simulink model "Antriebsstrangmodell_V1_4_n5_WHasym"  (R2019a)
(part 3 of 5)

  R_toBR_a(2.2)/LConn1 -- T_SH_a(2)/LConn1 -- C_SH_a(2)/LConn1 -- R_toBR_a(2.1)/RConn1 -- R_toRYO3(2)/RConn1
  R_toRSLTO(2)/RConn1 -- T_RYO(2)/LConn1 -- C_RYO(2)/LConn1 -- R_toSH(2)/LConn1 -- PV_RYO(2)/LConn1
  R_toRSL2(2)/RConn1 -- R_toRTO(2)/LConn1
  Thermal Reference32/LConn1 -- PV_RSL(2)/RConn2
  Thermal Reference33/LConn1 -- PV_RTO(2)/RConn2
  R_toRAGP(2)/LConn1 -- air-gap convection AGP to RSL (2)/RConn1
  Thermal Reference31/LConn1 -- PV_RYO(2)/RConn2
  R_toRAGP2(2)/LConn1 -- air-gap convection AGP to RTO (2)/RConn1
  R_toRTO(3)/RConn1 -- R_toRAGP(3)/RConn1 -- T_RSL(3)/LConn1 -- C_RSL(3)/LConn1 -- PV_RSL(3)/LConn1 -- R_toER(3.2)/LConn1 -- R_toER(3.1)/RConn1 -- R_toRYO(3)/LConn1
  C_RTO(3)/LConn1 -- T_RTO(3)/LConn1 -- PV_RTO(3)/LConn1 -- R_toRYO2(3)/LConn1 -- R_toRAGP2(3)/RConn1 -- R_toRSL2(3)/LConn1
  R_toRYO2(3)/RConn1 -- R_toRYO(3)/RConn1 -- R_toRSLTO(3)/LConn1
  R_toRSLTO(3)/RConn1 -- T_RYO(3)/LConn1 -- C_RYO(3)/LConn1 -- R_toSH(3)/LConn1 -- PV_RYO(3)/LConn1
  R_toRSL2(3)/RConn1 -- R_toRTO(3)/LConn1
  Thermal Reference35/LConn1 -- PV_RSL(3)/RConn2
  Thermal Reference36/LConn1 -- PV_RTO(3)/RConn2
  R_toRAGP(3)/LConn1 -- air-gap convection AGP to RSL (3)/RConn1
  Thermal Reference34/LConn1 -- PV_RYO(3)/RConn2
  R_toRAGP2(3)/LConn1 -- air-gap convection AGP to RTO (3)/RConn1
  R_toRTO(4)/RConn1 -- R_toRAGP(4)/RConn1 -- T_RSL(4)/LConn1 -- C_RSL(4)/LConn1 -- PV_RSL(4)/LConn1 -- R_toER(4.2)/LConn1 -- R_toER(4.1)/RConn1 -- R_toRYO(4)/LConn1
  C_RTO(4)/LConn1 -- T_RTO(4)/LConn1 -- PV_RTO(4)/LConn1 -- R_toRYO2(4)/LConn1 -- R_toRAGP2(4)/RConn1 -- R_toRSL2(4)/LConn1
  R_toRYO2(4)/RConn1 -- R_toRYO(4)/RConn1 -- R_toRSLTO(4)/LConn1
  R_toBR_a(4.2)/LConn1 -- T_SH_a(4)/LConn1 -- C_SH_a(4)/LConn1 -- R_toBR_a(4.1)/RConn1 -- R_toRYO3(4)/RConn1
  R_toRSLTO(4)/RConn1 -- T_RYO(4)/LConn1 -- C_RYO(4)/LConn1 -- R_toSH(4)/LConn1 -- PV_RYO(4)/LConn1
  R_toRSL2(4)/RConn1 -- R_toRTO(4)/LConn1
  Thermal Reference38/LConn1 -- PV_RSL(4)/RConn2
  Thermal Reference39/LConn1 -- PV_RTO(4)/RConn2
  R_toRAGP(4)/LConn1 -- air-gap convection AGP to RSL (4)/RConn1
  Thermal Reference37/LConn1 -- PV_RYO(4)/RConn2
  R_toRAGP2(4)/LConn1 -- air-gap convection AGP to RTO (4)/RConn1
  R_toRTO(5)/RConn1 -- R_toRAGP(5)/RConn1 -- T_RSL(5)/LConn1 -- C_RSL(5)/LConn1 -- PV_RSL(5)/LConn1 -- R_toER(5.2)/LConn1 -- R_toER(5.1)/RConn1 -- R_toRYO(5)/LConn1
  C_RTO(5)/LConn1 -- T_RTO(5)/LConn1 -- PV_RTO(5)/LConn1 -- R_toRYO2(5)/LConn1 -- R_toRAGP2(5)/RConn1 -- R_toRSL2(5)/LConn1
  R_toRYO(5)/RConn1 -- R_toRYO2(5)/RConn1 -- R_toRSLTO(5)/LConn1
  R_toBR_a(5.2)/LConn1 -- T_SH_a(5)/LConn1 -- C_SH_a(5)/LConn1 -- R_toBR_a(5.1)/RConn1 -- R_toRYO3(5)/RConn1
  R_toRSLTO(5)/RConn1 -- T_RYO(5)/LConn1 -- C_RYO(5)/LConn1 -- R_toSH(5)/LConn1 -- PV_RYO(5)/LConn1
  R_toRSL2(5)/RConn1 -- R_toRTO(5)/LConn1
  Thermal Reference41/LConn1 -- PV_RSL(5)/RConn2
  Thermal Reference42/LConn1 -- PV_RTO(5)/RConn2
  R_toRAGP(5)/LConn1 -- air-gap convection AGP to RSL (5)/RConn1
  Thermal Reference40/LConn1 -- PV_RYO(5)/RConn2
  R_toRAGP2(5)/LConn1 -- air-gap convection AGP to RTO (5)/RConn1
  R_toER(2.1)/LConn1 -- R_toER(1.2)/RConn1
  R_toER(2.2)/RConn1 -- R_toER(3.1)/LConn1
  R_toER(3.2)/RConn1 -- R_toER(4.1)/LConn1
  R_toER(4.2)/RConn1 -- R_toER(5.1)/LConn1
  C_ER(2)/LConn1 -- T_ER(2)/LConn1 -- R_toIA4(2)/RConn1 -- PV_ER(2)/LConn1 -- R_toIA3(2)/LConn1 -- R_toRSL(2.2)/LConn1 -- R_toRSL(2.1)/RConn1
  Thermal Reference6/LConn1 -- PV_ER(2)/RConn2
  C_ER(1)/LConn1 -- T_ER(1)/LConn1 -- R_toIA4(1)1/RConn1 -- R_toRSL(1.2)/LConn1 -- R_toIA3(1)/LConn1 -- PV_ER(1)/LConn1 -- R_toRSL(1.1)/RConn1
  Thermal Reference43/LConn1 -- PV_ER(1)/RConn2
  Thermal Reference5/LConn1 -- T_ER(1)/RConn1
  R_toEC_p(1.2)/RConn1 -- R_toEC_a(1.1)/LConn1
  R_toEC_p(2.2)/LConn1 -- C_HO_p(2)/LConn1 -- T_HO_p(2)/LConn1 -- R_toEC_p(2.1)/RConn1 -- R_toIA5(2)/LConn1 -- R_toWC_p(2)/RConn1
  R_toEC_p(2.1)/LConn1 -- R_toEC_a(5.2)/RConn1
  R_toHO2(2)/LConn1 -- R_toEC_p(2.2)/RConn1
  R_toBR2(2)/LConn1 -- T_EC(2)/LConn1 -- C_EC(2)/LConn1 -- R_toHO2(2)/RConn1 -- R_toIA7(2)/RConn1
  R_toBR2(1)/LConn1 -- R_toHO2(1)/RConn1 -- C_EC(1)/LConn1 -- R_toIA7(1)/LConn1 -- T_EC(1)/LConn1
  R_toHO2(1)/LConn1 -- R_toEC_p(1.1)/LConn1
  Thermal Reference4/LConn1 -- PV_BR(1.1)/RConn2
  R_toBR_p(1.2)/RConn1 -- R_toBR_a(1.1)/LConn1
  R_contactBR(1)/RConn1 -- PV_BR(1.2)/LConn1 -- R_toBR_p(1.1)/LConn1 -- Solver Configuration/RConn1
  R_toBR_a(2.2)/RConn1 -- R_toBR_a(3.1)/LConn1
  R_toBR_a(2.1)/LConn1 -- R_toBR_a(1.2)/RConn1
  R_toBR_a(3.2)/RConn1 -- R_toBR_a(4.1)/LConn1
  R_toBR_a(4.2)/RConn1 -- R_toBR_a(5.1)/LConn1
  R_toBR_a(5.2)/RConn1 -- R_toBR_p(2.1)/LConn1
  inner air convection EC to inner air (1)/LConn1 -- inner air convection WH to inner air (1.2)/LConn1 -- inner air convection HO to inner air (1)/LConn1 -- inner air convection WH to inner air (1.1)/LConn1 -- inner air convection WH to inner air (1.3)/LConn1 -- inner air convection ER to inner air (1.1)/LConn1 -- inner air convection SH to inner air (1)/LConn1 -- T_IA(1)/LConn1 -- PV_IA(1)/LConn1 -- inner air convection ER to inner air (1.2)/LConn1 -- inner air convection ER to inner air (1.3)/LConn1
  inner air convection EC to inner air (1)/LConn2 -- inner air convection HO to inner air (1)/LConn2 -- inner air convection WH to inner air (1.2)/LConn2 -- inner air convection WH to inner air (1.1)/LConn2 -- inner air convection WH to inner air (1.3)/LConn2 -- Simulink-PS Converter2/RConn1 -- inner air convection ER to inner air (1.1)/LConn2 -- inner air convection ER to inner air (1.2)/LConn2 -- inner air convection SH to inner air (1)/LConn2 -- inner air convection ER to inner air (1.3)/LConn2 -- inner air convection HO to inner air (2)/LConn2 -- inner air convection WH to inner air (2.2)/LConn2 -- inner air convection WH to inner air (2.1)/LConn2 -- inner air convection WH to inner air (2.3)/LConn2 -- inner air convection SH to inner air (2)/LConn2 -- inner air convection ER to inner air (2.2)/LConn2 -- inner air convection ER to inner air (2.1)/LConn2 -- inner air convection ER to inner air (2.3)/LConn2 -- inner air convection EC to inner air (2)/LConn2
  PV_ER(2)/RConn1 -- Simulink-PS Converter14/RConn1
  Simulink-PS Converter19/RConn1 -- PV_BR(2.2)/RConn1 -- PV_BR(2.1)/RConn1
  Simulink-PS Converter9/RConn1 -- PV_BR(1.2)/RConn1 -- PV_BR(1.1)/RConn1
  Thermal Reference45/LConn1 -- T_SSL(5)/RConn1
  Thermal Reference46/LConn1 -- T_SSL(4)/RConn1
  R_toSSL(2.2)/RConn1 -- inner air convection WH to inner air (2.1)/RConn1
  C_WH(2)/LConn1 -- T_WH(2)/LConn1 -- R_toIA2(2)/LConn1 -- PV_WH(2)/LConn1 -- R_toSSL(2.2)/LConn1 -- R_toIA(2)/RConn1 -- R_toSSL(2.1)/RConn1
  R_toWH(1.1)/LConn1 -- R_toSSL(1.2)/RConn1
  R_contactHO (1)/RConn1 -- R_toHO(1)/LConn1
  R_toHO(2)/LConn1 -- R_contactHO (2)/RConn1
  R_toHO(5)/LConn1 -- R_contactHO (5)/RConn1
  R_toRSL(1.1)/LConn1 -- inner air convection ER to inner air (1.1)/RConn1
  R_toER(1.1)/LConn1 -- R_toRSL(1.2)/RConn1
  R_toRSL(2.1)/LConn1 -- R_toER(5.2)/RConn1
  R_toRSL(2.2)/RConn1 -- inner air convection ER to inner air (2.1)/RConn1
  inner air convection ER to inner air (1.2)/RConn1 -- R_toIA3(1)/RConn1
  inner air convection ER to inner air (1.3)/RConn1 -- R_toIA4(1)1/LConn1
  inner air convection ER to inner air (2.2)/RConn1 -- R_toIA3(2)/RConn1
  inner air convection ER to inner air (2.3)/RConn1 -- R_toIA4(2)/LConn1
  air-gap convection AGP to RSL (2)/LConn1 -- air-gap convection AGP to SSL (2)/LConn1 -- T_AGP(2)/LConn1 -- air-gap convection AGP to STO (2)/LConn1 -- PV_AGP(2)/LConn1 -- air-gap convection AGP to RTO (2)/LConn1
  air-gap convection AGP to RSL (4)/LConn1 -- air-gap convection AGP to SSL (4)/LConn1 -- T_AGP(4)/LConn1 -- air-gap convection AGP to STO (4)/LConn1 -- PV_AGP(4)/LConn1 -- air-gap convection AGP to RTO (4)/LConn1
  air-gap convection AGP to STO (5)/LConn1 -- PV_AGP(5)/LConn1 -- T_AGP(5)/LConn1 -- air-gap convection AGP to RSL (5)/LConn1 -- air-gap convection AGP to SSL (5)/LConn1 -- air-gap convection AGP to RTO (5)/LConn1
  Thermal Reference44/LConn1 -- PV_AGP(2)/RConn2
  Thermal Reference47/LConn1 -- PV_AGP(3)/RConn2
  Thermal Reference48/LConn1 -- PV_AGP(4)/RConn2
  Thermal Reference49/LConn1 -- PV_AGP(5)/RConn2
  R_toEC_p(1.2)/LConn1 -- R_toIA5(1)/LConn1 -- R_toWC_p(1)/RConn1 -- C_HO_p(1)/LConn1 -- T_HO_p(1)/LConn1 -- R_toEC_p(1.1)/RConn1
  inner air convection WH to inner air (2.2)/RConn1 -- R_toIA(2)/LConn1
  R_toIA2(2)/RConn1 -- inner air convection WH to inner air (2.3)/RConn1
  R_toIA2(1)/RConn1 -- inner air convection WH to inner air (1.3)/RConn1
  R_toSSL(1.1)/LConn1 -- inner air convection WH to inner air (1.1)/RConn1
  inner air convection WH to inner air (1.2)/RConn1 -- R_toIA(1)/LConn1
  Convection HO to coolant (1)/LConn1 -- R_toWC_p(1)/LConn1
  Convection HO to coolant (7)/LConn1 -- R_toWC_p(2)/LConn1
  R_toIA5(1)/RConn1 -- inner air convection HO to inner air (1)/RConn1
  inner air convection HO to inner air (2)/RConn1 -- R_toIA5(2)/RConn1
  C_SH_a(1)/LConn1 -- R_toBR_a(1.2)/LConn1 -- R_toBR_a(1.1)/RConn1 -- R_toRYO3(1)/RConn1 -- T_SH_a(1)/LConn1
  R_toBR_a(3.2)/LConn1 -- T_SH_a(3)/LConn1 -- C_SH_a(3)/LConn1 -- R_toBR_a(3.1)/RConn1 -- R_toRYO3(3)/RConn1
  R_toIA6(1)/LConn1 -- inner air convection SH to inner air (1)/RConn1
  R_toIA6(1)/RConn1 -- C_SH_p(1)/LConn1 -- R_toBR_p(1.2)/LConn1 -- T_SH_p(1)/LConn1 -- R_toBR_p(1.1)/RConn1
  R_toIA6(2)/RConn1 -- T_SH_p(2)/LConn1 -- R_toBR_p(2.2)/LConn1 -- R_toBR_p(2.1)/RConn1 -- C_SH_p(2)/LConn1
  R_toIA6(2)/LConn1 -- inner air convection SH to inner air (2)/RConn1
  Thermal Reference50/LConn1 -- PV_BR(1.2)/RConn2
  PV_BR(1.1)/LConn1 -- R_toBR2(1)/RConn1 -- R_contactBR(1)/LConn1
  Thermal Reference51/LConn1 -- PV_BR(2.2)/RConn2
  R_toBR2(2)/RConn1 -- PV_BR(2.1)/LConn1 -- R_contactBR(2)/LConn1
  R_toIA7(1)/RConn1 -- inner air convection EC to inner air (1)/RConn1
  R_toIA7(2)/LConn1 -- inner air convection EC to inner air (2)/RConn1
  Thermal Reference53/LConn1 -- T_SSL(1)/RConn1
  Thermal Reference54/LConn1 -- T_SSL(2)/RConn1
  Simulink-PS Converter32/RConn1 -- PV_RYO(5)/RConn1
  PV_RYO(4)/RConn1 -- Simulink-PS Converter31/RConn1
  PV_RYO(3)/RConn1 -- Simulink-PS Converter30/RConn1
  PV_RYO(2)/RConn1 -- Simulink-PS Converter29/RConn1
  PV_RYO(1)/RConn1 -- Simulink-PS Converter16/RConn1
  Thermal Reference55/LConn1 -- T_RYO(1)/RConn1
  Thermal Reference56/LConn1 -- T_RYO(2)/RConn1
  Thermal Reference57/LConn1 -- T_RYO(3)/RConn1
  Thermal Reference58/LConn1 -- T_RYO(4)/RConn1
  Thermal Reference59/LConn1 -- T_RYO(5)/RConn1
  PS-Simulink Converter11/LConn1 -- T_RYO(5)/RConn2
  PS-Simulink Converter12/LConn1 -- T_RYO(4)/RConn2
  PS-Simulink Converter13/LConn1 -- T_RYO(3)/RConn2
  PS-Simulink Converter14/LConn1 -- T_RYO(2)/RConn2
  PS-Simulink Converter15/LConn1 -- T_RYO(1)/RConn2
  Simulink-PS Converter37/RConn1 -- PV_RTO(5)/RConn1
  Simulink-PS Converter36/RConn1 -- PV_RTO(4)/RConn1
  Simulink-PS Converter35/RConn1 -- PV_RTO(3)/RConn1
  Simulink-PS Converter34/RConn1 -- PV_RTO(2)/RConn1
  Simulink-PS Converter33/RConn1 -- PV_RTO(1)/RConn1
  Thermal Reference60/LConn1 -- T_RTO(1)/RConn1
  Thermal Reference61/LConn1 -- T_RTO(2)/RConn1
  Thermal Reference62/LConn1 -- T_RTO(3)/RConn1
  Thermal Reference63/LConn1 -- T_RTO(4)/RConn1
  Thermal Reference64/LConn1 -- T_RTO(5)/RConn1
  PS-Simulink Converter16/LConn1 -- T_RTO(5)/RConn2
  PS-Simulink Converter17/LConn1 -- T_RTO(4)/RConn2
  PS-Simulink Converter18/LConn1 -- T_RTO(3)/RConn2
  PS-Simulink Converter19/LConn1 -- T_RTO(2)/RConn2
  PS-Simulink Converter20/LConn1 -- T_RTO(1)/RConn2
  Simulink-PS Converter41/RConn1 -- PV_RSL(5)/RConn1
  Simulink-PS Converter40/RConn1 -- PV_RSL(4)/RConn1
  Simulink-PS Converter39/RConn1 -- PV_RSL(3)/RConn1
  Simulink-PS Converter38/RConn1 -- PV_RSL(2)/RConn1
  Simulink-PS Converter18/RConn1 -- PV_RSL(1)/RConn1
  Thermal Reference65/LConn1 -- T_RSL(2)/RConn1
  Thermal Reference66/LConn1 -- T_RSL(1)/RConn1
  Thermal Reference67/LConn1 -- T_RSL(4)/RConn1
  Thermal Reference68/LConn1 -- T_RSL(5)/RConn1
  PS-Simulink Converter21/LConn1 -- T_RSL(5)/RConn2
  PS-Simulink Converter22/LConn1 -- T_RSL(4)/RConn2
  PS-Simulink Converter23/LConn1 -- T_RSL(3)/RConn2
  PS-Simulink Converter24/LConn1 -- T_RSL(2)/RConn2
  T_RSL(1)/RConn2 -- PS-Simulink Converter25/LConn1
  Simulink-PS Converter13/RConn1 -- PV_ER(1)/RConn1
  PS-Simulink Converter5/LConn1 -- T_ER(2)/RConn2
  PS-Simulink Converter26/LConn1 -- T_ER(1)/RConn2
  Simulink-PS Converter6/RConn1 -- air-gap convection AGP to RSL (5)/LConn2 -- air-gap convection AGP to RTO (5)/LConn2 -- air-gap convection AGP to RSL (4)/LConn2 -- air-gap convection AGP to RTO (4)/LConn2 -- air-gap convection AGP to RSL (3)/LConn2 -- air-gap convection AGP to RTO (3)/LConn2 -- air-gap convection AGP to RSL (2)/LConn2 -- air-gap convection AGP to RTO (2)/LConn2 -- air-gap convection AGP to RSL (1)/LConn2 -- air-gap convection AGP to RTO (1)/LConn2 -- air-gap convection AGP to STO (1)/LConn2 -- air-gap convection AGP to SSL (2)/LConn2 -- air-gap convection AGP to STO (3)/LConn2 -- air-gap convection AGP to SSL (4)/LConn2 -- air-gap convection AGP to STO (5)/LConn2 -- air-gap convection AGP to SSL (5)/LConn2 -- air-gap convection AGP to STO (4)/LConn2 -- air-gap convection AGP to SSL (3)/LConn2 -- air-gap convection AGP to STO (2)/LConn2 -- air-gap convection AGP to SSL (1)/LConn2
  Thermal Reference69/LConn1 -- T_AGP(1)/RConn1
  Thermal Reference70/LConn1 -- T_AGP(2)/RConn1
  Thermal Reference71/LConn1 -- T_AGP(3)/RConn1
  Thermal Reference72/LConn1 -- T_AGP(4)/RConn1
  Thermal Reference73/LConn1 -- T_AGP(5)/RConn1
  PS-Simulink Converter6/LConn1 -- T_AGP(5)/RConn2
  PS-Simulink Converter27/LConn1 -- T_AGP(4)/RConn2
  PS-Simulink Converter29/LConn1 -- T_AGP(2)/RConn2
  PS-Simulink Converter28/LConn1 -- T_AGP(3)/RConn2
  T_AGP(1)/RConn2 -- PS-Simulink Converter30/LConn1
  Simulink-PS Converter12/RConn1 -- PV_AGP(1)/RConn1
  Simulink-PS Converter42/RConn1 -- PV_AGP(2)/RConn1
  PV_AGP(3)/RConn1 -- Simulink-PS Converter43/RConn1
  PV_AGP(4)/RConn1 -- Simulink-PS Converter44/RConn1
  PV_AGP(5)/RConn1 -- Simulink-PS Converter45/RConn1
  inner air convection EC to inner air (2)/LConn1 -- inner air convection HO to inner air (2)/LConn1 -- inner air convection WH to inner air (2.2)/LConn1 -- inner air convection WH to inner air (2.1)/LConn1 -- inner air convection WH to inner air (2.3)/LConn1 -- inner air convection ER to inner air (2.1)/LConn1 -- T_IA(2)/LConn1 -- inner air convection SH to inner air (2)/LConn1 -- PV_IA(2)/LConn1 -- inner air convection ER to inner air (2.2)/LConn1 -- inner air convection ER to inner air (2.3)/LConn1
  Thermal Reference52/LConn1 -- T_WH(1)/RConn1
  T_WH(1)/RConn2 -- PS-Simulink Converter8/LConn1
  Simulink-PS Converter7/RConn1 -- PV_SSL(1)/RConn1
  Simulink-PS Converter8/RConn1 -- PV_SSL(2)/RConn1
  PV_SSL(3)/RConn1 -- Simulink-PS Converter10/RConn1
  PV_SSL(4)/RConn1 -- Simulink-PS Converter11/RConn1
  PV_SSL(5)/RConn1 -- Simulink-PS Converter1/RConn1
  PS-Simulink Converter35/LConn1 -- T_SSL(5)/RConn2
  T_SSL(4)/RConn2 -- PS-Simulink Converter31/LConn1
  PS-Simulink Converter32/LConn1 -- T_SSL(3)/RConn2
  PS-Simulink Converter33/LConn1 -- T_SSL(2)/RConn2
  PS-Simulink Converter34/LConn1 -- T_SSL(1)/RConn2
  Thermal Reference74/LConn1 -- T_STO(1)/RConn1
  Thermal Reference75/LConn1 -- T_STO(2)/RConn1
  Thermal Reference76/LConn1 -- T_STO(3)/RConn1
  Thermal Reference77/LConn1 -- T_STO(4)/RConn1
  Thermal Reference78/LConn1 -- T_STO(5)/RConn1
  Simulink-PS Converter5/RConn1 -- PV_WH(2)/RConn1
  Simulink-PS Converter20/RConn1 -- PV_WH(1)/RConn1
  Simulink-PS Converter15/RConn1 -- PV_STO(1)/RConn1
  Simulink-PS Converter21/RConn1 -- PV_STO(2)/RConn1
  Simulink-PS Converter22/RConn1 -- PV_STO(5)/RConn1
  Simulink-PS Converter24/RConn1 -- PV_STO(4)/RConn1
  PV_STO(3)/RConn1 -- Simulink-PS Converter23/RConn1
  PS-Simulink Converter10/LConn1 -- T_STO(5)/RConn2
  PS-Simulink Converter2/LConn1 -- T_STO(4)/RConn2
  PS-Simulink Converter3/LConn1 -- T_STO(3)/RConn2
  PS-Simulink Converter7/LConn1 -- T_STO(2)/RConn2
  PS-Simulink Converter9/LConn1 -- T_STO(1)/RConn2
  Thermal Reference79/LConn1 -- T_SYO(1)/RConn1
  Thermal Reference80/LConn1 -- T_SYO(2)/RConn1
  Thermal Reference81/LConn1 -- T_SYO(3)/RConn1
  Thermal Reference82/LConn1 -- T_SYO(4)/RConn1
  Thermal Reference83/LConn1 -- T_SYO(5)/RConn1
  Simulink-PS Converter28/RConn1 -- PV_SYO(5)/RConn1
  Simulink-PS Converter26/RConn1 -- PV_SYO(4)/RConn1
  Simulink-PS Converter27/RConn1 -- PV_SYO(3)/RConn1
  Simulink-PS Converter25/RConn1 -- PV_SYO(2)/RConn1
  Simulink-PS Converter17/RConn1 -- PV_SYO(1)/RConn1
  PS-Simulink Converter36/LConn1 -- T_SYO(5)/RConn2
  PS-Simulink Converter40/LConn1 -- T_SYO(1)/RConn2
  PS-Simulink Converter37/LConn1 -- T_SYO(4)/RConn2
  PS-Simulink Converter39/LConn1 -- T_SYO(2)/RConn2
  PS-Simulink Converter38/LConn1 -- T_SYO(3)/RConn2
  Thermal Reference84/LConn1 -- PV_IA(1)/RConn2
  Simulink-PS Converter46/RConn1 -- PV_IA(1)/RConn1
  Thermal Reference86/LConn1 -- T_IA(1)/RConn1
  Thermal Reference85/LConn1 -- PV_IA(2)/RConn2
  Thermal Reference87/LConn1 -- T_IA(2)/RConn1
  PS-Simulink Converter41/LConn1 -- T_IA(2)/RConn2
  Simulink-PS Converter47/RConn1 -- PV_IA(2)/RConn1
  T_IA(1)/RConn2 -- PS-Simulink Converter42/LConn1
  Thermal Reference88/LConn1 -- T_SH_a(1)/RConn1
  Thermal Reference89/LConn1 -- T_SH_a(2)/RConn1
  Thermal Reference90/LConn1 -- T_SH_a(3)/RConn1
  Thermal Reference91/LConn1 -- T_SH_a(4)/RConn1
  Thermal Reference92/LConn1 -- T_SH_a(5)/RConn1
  Thermal Reference93/LConn1 -- T_SH_p(2)/RConn1
  Thermal Reference94/LConn1 -- T_SH_p(1)/RConn1
  PS-Simulink Converter47/LConn1 -- T_SH_p(2)/RConn2
  PS-Simulink Converter46/LConn1 -- T_SH_a(5)/RConn2
  PS-Simulink Converter45/LConn1 -- T_SH_a(4)/RConn2
  PS-Simulink Converter44/LConn1 -- T_SH_a(3)/RConn2
  PS-Simulink Converter43/LConn1 -- T_SH_a(2)/RConn2
  PS-Simulink Converter49/LConn1 -- T_SH_a(1)/RConn2
  PS-Simulink Converter48/LConn1 -- T_SH_p(1)/RConn2
  Thermal Reference95/LConn1 -- T_HO_a(1)/RConn1
  Thermal Reference96/LConn1 -- T_HO_a(2)/RConn1
  Thermal Reference97/LConn1 -- T_HO_p(1)/RConn1
  Thermal Reference98/LConn1 -- T_HO_a(3)/RConn1
  Thermal Reference99/LConn1 -- T_HO_a(4)/RConn1
  Thermal Reference100/LConn1 -- T_HO_a(5)/RConn1
  Thermal Reference101/LConn1 -- T_HO_p(2)/RConn1
  PS-Simulink Converter55/LConn1 -- T_HO_p(2)/RConn2
  PS-Simulink Converter56/LConn1 -- T_HO_a(5)/RConn2
  PS-Simulink Converter50/LConn1 -- T_HO_a(4)/RConn2
  PS-Simulink Converter51/LConn1 -- T_HO_a(3)/RConn2
  PS-Simulink Converter52/LConn1 -- T_HO_a(2)/RConn2
  PS-Simulink Converter53/LConn1 -- T_HO_a(1)/RConn2
  PS-Simulink Converter54/LConn1 -- T_HO_p(1)/RConn2
  Thermal Reference102/LConn1 -- T_EC(2)/RConn1
  Thermal Reference103/LConn1 -- T_EC(1)/RConn1
  PS-Simulink Converter57/LConn1 -- T_EC(2)/RConn2
  PS-Simulink Converter58/LConn1 -- T_EC(1)/RConn2
  C_WH(1)/LConn1 -- T_WH(1)/LConn1 -- R_toSSL(1.2)/LConn1 -- R_toIA2(1)/LConn1 -- PV_WH(1)/LConn1 -- R_toIA(1)/RConn1 -- R_toSSL(1.1)/RConn1
  Variable Thermal Resistance1/LConn1 -- Konvektion Radiator an Umgebungsluft (keine Geschw.Abhängigkeit)/LConn1
  R_toSYO3(1)/RConn1 -- R_contactHO (1)/LConn1
  R_toSYO3(2)/RConn1 -- R_contactHO (2)/LConn1
  R_toSYO3(3)/RConn1 -- R_contactHO (3)/LConn1
  R_toSYO3(4)/RConn1 -- R_contactHO (4)/LConn1
  R_toSYO3(5)/RConn1 -- R_contactHO (5)/LConn1
  R_toSH(1)/RConn1 -- R_toRYO3(1)/LConn1
  R_toSH(2)/RConn1 -- R_toRYO3(2)/LConn1
  R_toSH(3)/RConn1 -- R_toRYO3(3)/LConn1
  R_toSH(4)/RConn1 -- R_toRYO3(4)/LConn1
  R_toRYO3(5)/LConn1 -- R_toSH(5)/RConn1
  PV_AGP(1)/LConn1 -- air-gap convection AGP to STO (1)/LConn1 -- air-gap convection AGP to RSL (1)/LConn1 -- air-gap convection AGP to SSL (1)/LConn1 -- T_AGP(1)/LConn1 -- air-gap convection AGP to RTO (1)/LConn1
